simulink model "Heli_Voltage_Set"  (R2015b)
settings: Solver=FixedStepDiscrete  StartTime=0.0  StopTime=inf  FixedStep=0.01  RelTol=1e-3
values from neighbouring files (symbols this model uses):
  D2R = pi/180.0    (= 0.0174532925199)    [Heli_Setup.m]
  ELEV_START = -24.25    [Heli_Setup.m]
  K_CABLE = 5    [Heli_Setup.m]
  K_DAQ = 10    [Heli_Setup.m]
  KE_C2D = -360/4096    (= -0.087890625)    [Heli_Setup.m]
  R2D = 180/pi    (= 57.2957795131)    [Heli_Setup.m]
  VSUM_MAX = 36    [Heli_Setup.m]
undefined symbols (not defined in the file or in its folder): HIL
libraries: quarc_library x4, simulink x1
settings Model: SimulationMode=external  ExtModeTrigDuration=10000  Creator=Admin  LastModifiedBy=AER509
settings SolverCC: PositivePriorityOrder=on
settings DataIOCC: LimitDataPoints=off  SaveFormat=StructureWithTime
settings OptimizationCC: ExpressionDepthLimit=2147483647
settings DebuggingCC: UnderspecifiedInitializationDetection=Classic  MergeDetectMultiDrivingBlocksExec=none  SolverPrmCheckMsg=warning  StateNameClashWarn=warning
settings HardwareCC: ProdBitPerPointer=32  ProdLargestAtomicFloat=None  ProdIntDivRoundTo=Undefined  ProdEndianess=Unspecified  ProdWordSize=32  ProdHWDeviceType=32-bit Generic
settings RTWCC: SystemTargetFile=quarc_win64.tlc  TemplateMakefile=quarc_default_tmf  Description=QUARC Win64 Target
settings STFCustomTargetCC: CombineOutputUpdateFcns=on  GRTInterface=off
settings GRTTargetCC: ParMdlRefBuildCompliant=off  CompOptLevelCompliant=off  GeneratePreprocessorConditionals=Disable all  MatFileLogging=off  UseToolchainInfoCompliant=off  ExtMode=on  ExtModeMexFile=quarc_comm
settings ConfigComp: CovModelRefEnable=Off

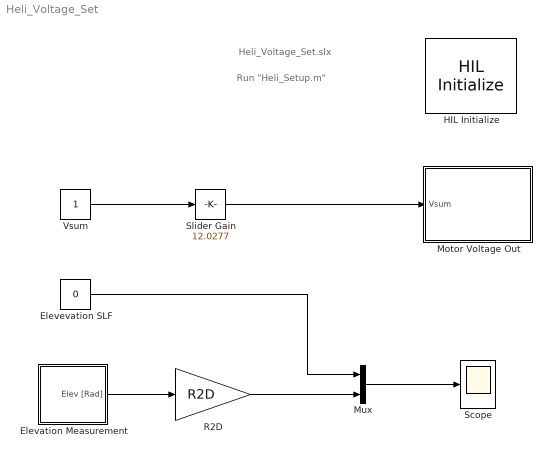
== system Heli_Voltage_Set ==
  note: Run "Heli_Setup.m"
  note: Heli_Voltage_Set.slx
  Elevation Measurement : Subsystem
  Elevevation SLF : Constant  Value=0
  HIL Initialize : quarc_library/Data Acquisition/Generic/Configuration/HIL Initialize  Priority=-99  object_name=HIL-1  board_type=q4  board_number=0  board_options=""  exclusive=off  active=off  hardware_clocks=[0:1]  clock_modes=[0 0]  initial_clock_frequencies=[]  set_clock_params_at_start=on  set_clock_params_at_switch_in=off  set_clock_frequencies_at_start=off  set_clock_frequencies_at_switch_in=off  analog_input_channels=[0:3]  analog_input_maximums=10  analog_input_minimums=-10  set_analog_input_params_at_start=off  set_analog_input_params_at_switch_in=off  analog_output_channels=[0:3]  analog_output_maximums=[10]  analog_output_minimums=[-10]  initial_analog_outputs=[0]  final_analog_outputs=[0]  watchdog_analog_outputs=0  set_analog_output_params_at_start=on  set_analog_output_params_at_switch_in=off  set_analog_outputs_at_start=on  set_analog_outputs_at_switch_in=off  set_analog_outputs_at_terminate=on  set_analog_outputs_at_switch_out=off  set_analog_outputs_on_watchdog=off  digital_input_channels=[]  digital_output_channels=[]  digital_output_configuration=[]  initial_digital_outputs=[1]  final_digital_outputs=[1]  watchdog_digital_outputs=[2]  set_digital_output_params_at_start=off  set_digital_output_params_at_switch_in=off  set_digital_outputs_at_start=on  set_digital_outputs_at_switch_in=off  set_digital_outputs_at_terminate=on  set_digital_outputs_at_switch_out=off  set_digital_outputs_on_watchdog=off  encoder_channels=[0:3]  quadrature=[4]  encoder_filter_frequency=(1/60e-9)/1  initial_encoder_counts=[0]  set_encoder_params_at_start=on  set_encoder_params_at_switch_in=off  set_encoder_counts_at_start=on  set_encoder_counts_at_switch_in=off  pwm_channels=[]  pwm_modes=[0]  pwm_frequency=(1/60e-9)/1024  pwm_configuration=[]  pwm_alignment=[]  pwm_polarity=[]  pwm_leading_deadband=[]  pwm_trailing_deadband=[]  initial_pwm_outputs=[0]  final_pwm_outputs=[0]  watchdog_pwm_outputs=[]  set_pwm_params_at_start=on  set_pwm_params_at_switch_in=off  set_pwm_outputs_at_start=on  set_pwm_outputs_at_switch_in=off  set_pwm_outputs_at_terminate=on  set_pwm_outputs_at_switch_out=off  set_pwm_outputs_on_watchdog=off  other_output_channels=[]  initial_other_outputs=[]  final_other_outputs=[]  watchdog_other_outputs=[]  set_other_outputs_at_start=off  set_other_outputs_at_switch_in=off  set_other_outputs_at_terminate=off  set_other_outputs_at_switch_out=off  set_other_outputs_on_watchdog=off
  Motor Voltage Out : Subsystem
  Mux : Mux  Inputs=2
  R2D : Gain  Gain=R2D
  Scope : Scope
  Slider Gain : simulink/Math Operations/Slider Gain  low=0  gain=12.0277  high=30
  Vsum : Constant
  wires:
  Elevation Measurement/1(Elev [Rad]) -> R2D/1
  Vsum/1 -> Slider Gain/1
  Slider Gain/1 -> Motor Voltage Out/1(Vsum)
  Mux/1 -> Scope/1
  Elevevation SLF/1 -> Mux/1
  R2D/1 -> Mux/2

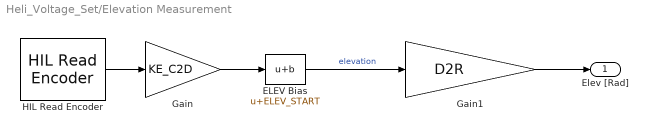
== system Heli_Voltage_Set/Elevation Measurement ==
  ELEV Bias : Bias  Bias=ELEV_START
  Gain : Gain  Gain=KE_C2D
  Gain1 : Gain  Gain=D2R
  HIL Read Encoder : quarc_library/Data Acquisition/Generic/Immediate I//O/HIL Read Encoder  object_name=HIL-1  channels=3  sample_time=qc_get_step_size  active=on  vector_output=off  data_type_mode=Inherit via back propagation  data_type=double
  Elev [Rad] : Outport
  wires:
  HIL Read Encoder/1 -> Gain/1
  Gain/1 -> ELEV Bias/1
  ELEV Bias/1 -> Gain1/1  "elevation"
  Gain1/1 -> Elev [Rad]/1

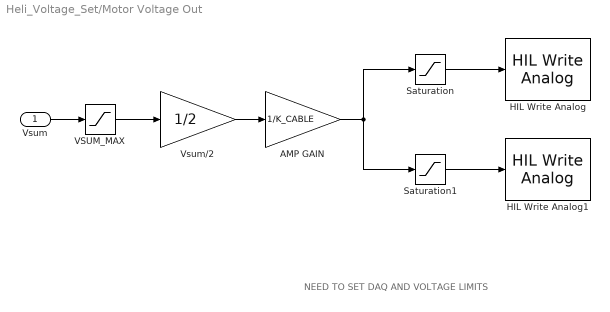
== system Heli_Voltage_Set/Motor Voltage Out ==
  note: NEED TO SET DAQ AND VOLTAGE LIMITS
  Vsum : Inport
  AMP GAIN : Gain  Gain=1/K_CABLE
  HIL Write Analog : quarc_library/Data Acquisition/Generic/Immediate I//O/HIL Write Analog  object_name=HIL-1  channels=2  sample_time=-1  active=off  vector_input=off
  HIL Write Analog1 : quarc_library/Data Acquisition/Generic/Immediate I//O/HIL Write Analog  object_name=HIL-1  channels=3  sample_time=-1  active=off  vector_input=off
  Saturation : Saturate  UpperLimit=K_DAQ  LowerLimit=-K_DAQ
  Saturation1 : Saturate  UpperLimit=K_DAQ  LowerLimit=-K_DAQ
  VSUM_MAX : Saturate  UpperLimit=VSUM_MAX  LowerLimit=0
  Vsum/2 : Gain  Gain=1/2
  wires:
  Vsum/1 -> VSUM_MAX/1
  AMP GAIN/1 -> Saturation/1, Saturation1/1
  Saturation/1 -> HIL Write Analog/1
  Saturation1/1 -> HIL Write Analog1/1
  Vsum/2/1 -> AMP GAIN/1
  VSUM_MAX/1 -> Vsum/2/1
